simulink library "csc_rtc_rts_collection_lib"  (R2014b)
settings: Solver=ode45  StartTime=0.0  StopTime=10.0  RelTol=1e-3
libraries: csu_exr_execute_rts_lib x11, util_info_lib x1
settings Model: Creator=jimkaidy  LastModifiedBy=jimkaidy

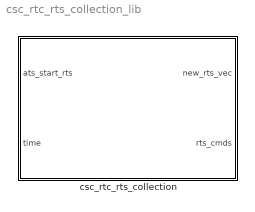
== system csc_rtc_rts_collection_lib ==
  csc_rtc_rts_collection : Subsystem
      mask Display: color('blue');text(0.05, 0.02, 'MoonEx', 'HorizontalAlignment', 'Left', 'VerticalAlignment', 'Bottom');color('red');text(0.95, 0.02, 'Autogenerated', 'HorizontalAlignment', 'Right', 'VerticalAlignment', 'Bottom');

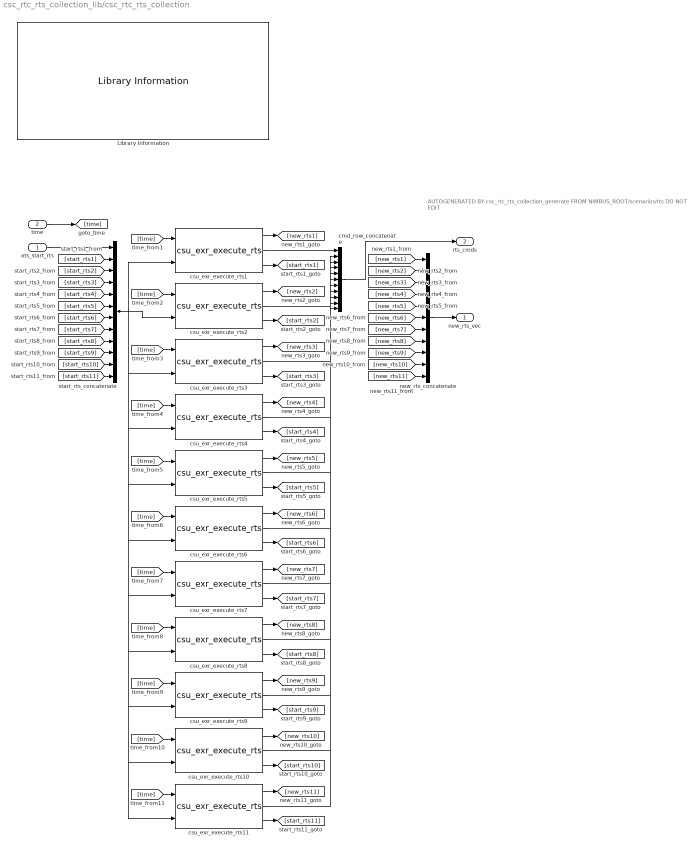
== system csc_rtc_rts_collection_lib/csc_rtc_rts_collection ==
  note: AUTOGENERATED BY csc_rtc_rts_collection_generate FROM
      | NIMBUS_ROOT/scenarios/rts
      | DO NOT EDIT
  ats_start_rts : Inport
  time : Inport  Port=2
  Library Information : util_info_lib/Library Information  owner='escrane'
  cmd_row_concatenate : Concatenate  NumInputs=11  Mode=Multidimensional array
  csu_exr_execute_rts1 : csu_exr_execute_rts_lib/csu_exr_execute_rts  rts_id=10  rts_tbl_cmd_time=sc_rts010_cmd_time  rts_tbl_cmd_data=sc_rts010_cmd_data
  csu_exr_execute_rts10 : csu_exr_execute_rts_lib/csu_exr_execute_rts  rts_id=52  rts_tbl_cmd_time=sc_rts052_cmd_time  rts_tbl_cmd_data=sc_rts052_cmd_data
  csu_exr_execute_rts11 : csu_exr_execute_rts_lib/csu_exr_execute_rts  rts_id=81  rts_tbl_cmd_time=sc_rts081_cmd_time  rts_tbl_cmd_data=sc_rts081_cmd_data
  csu_exr_execute_rts2 : csu_exr_execute_rts_lib/csu_exr_execute_rts  rts_id=12  rts_tbl_cmd_time=sc_rts012_cmd_time  rts_tbl_cmd_data=sc_rts012_cmd_data
  csu_exr_execute_rts3 : csu_exr_execute_rts_lib/csu_exr_execute_rts  rts_id=13  rts_tbl_cmd_time=sc_rts013_cmd_time  rts_tbl_cmd_data=sc_rts013_cmd_data
  csu_exr_execute_rts4 : csu_exr_execute_rts_lib/csu_exr_execute_rts  rts_id=14  rts_tbl_cmd_time=sc_rts014_cmd_time  rts_tbl_cmd_data=sc_rts014_cmd_data
  csu_exr_execute_rts5 : csu_exr_execute_rts_lib/csu_exr_execute_rts  rts_id=15  rts_tbl_cmd_time=sc_rts015_cmd_time  rts_tbl_cmd_data=sc_rts015_cmd_data
  csu_exr_execute_rts6 : csu_exr_execute_rts_lib/csu_exr_execute_rts  rts_id=1  rts_tbl_cmd_time=sc_rts001_cmd_time  rts_tbl_cmd_data=sc_rts001_cmd_data
  csu_exr_execute_rts7 : csu_exr_execute_rts_lib/csu_exr_execute_rts  rts_id=40  rts_tbl_cmd_time=sc_rts040_cmd_time  rts_tbl_cmd_data=sc_rts040_cmd_data
  csu_exr_execute_rts8 : csu_exr_execute_rts_lib/csu_exr_execute_rts  rts_id=50  rts_tbl_cmd_time=sc_rts050_cmd_time  rts_tbl_cmd_data=sc_rts050_cmd_data
  csu_exr_execute_rts9 : csu_exr_execute_rts_lib/csu_exr_execute_rts  rts_id=51  rts_tbl_cmd_time=sc_rts051_cmd_time  rts_tbl_cmd_data=sc_rts051_cmd_data
  new_rts_concatenate : Concatenate  NumInputs=11
  start_rts_concatenate : Concatenate  NumInputs=12
  new_rts_vec : Outport
  rts_cmds : Outport  Port=2
  wires:
  time/1 -> [time]
  ats_start_rts/1 -> start_rts_concatenate/1
  new_rts_concatenate/1 -> new_rts_vec/1
  [start_rts1] -> start_rts_concatenate/2
  [new_rts1] -> new_rts_concatenate/1
  [time] -> csu_exr_execute_rts1/1
  csu_exr_execute_rts1/1 -> [new_rts1]
  csu_exr_execute_rts1/3 -> [start_rts1]
  [start_rts2] -> start_rts_concatenate/3
  [new_rts2] -> new_rts_concatenate/2
  [time] -> csu_exr_execute_rts2/1
  csu_exr_execute_rts2/1 -> [new_rts2]
  csu_exr_execute_rts2/3 -> [start_rts2]
  [start_rts3] -> start_rts_concatenate/4
  [new_rts3] -> new_rts_concatenate/3
  [time] -> csu_exr_execute_rts3/1
  csu_exr_execute_rts3/1 -> [new_rts3]
  csu_exr_execute_rts3/3 -> [start_rts3]
  [start_rts4] -> start_rts_concatenate/5
  [new_rts4] -> new_rts_concatenate/4
  [time] -> csu_exr_execute_rts4/1
  csu_exr_execute_rts4/1 -> [new_rts4]
  csu_exr_execute_rts4/3 -> [start_rts4]
  [start_rts5] -> start_rts_concatenate/6
  [new_rts5] -> new_rts_concatenate/5
  [time] -> csu_exr_execute_rts5/1
  csu_exr_execute_rts5/1 -> [new_rts5]
  csu_exr_execute_rts5/3 -> [start_rts5]
  [start_rts6] -> start_rts_concatenate/7
  [new_rts6] -> new_rts_concatenate/6
  [time] -> csu_exr_execute_rts6/1
  csu_exr_execute_rts6/1 -> [new_rts6]
  csu_exr_execute_rts6/3 -> [start_rts6]
  [start_rts7] -> start_rts_concatenate/8
  [new_rts7] -> new_rts_concatenate/7
  [time] -> csu_exr_execute_rts7/1
  csu_exr_execute_rts7/1 -> [new_rts7]
  csu_exr_execute_rts7/3 -> [start_rts7]
  [start_rts8] -> start_rts_concatenate/9
  [new_rts8] -> new_rts_concatenate/8
  [time] -> csu_exr_execute_rts8/1
  csu_exr_execute_rts8/1 -> [new_rts8]
  csu_exr_execute_rts8/3 -> [start_rts8]
  [start_rts9] -> start_rts_concatenate/10
  [new_rts9] -> new_rts_concatenate/9
  [time] -> csu_exr_execute_rts9/1
  csu_exr_execute_rts9/1 -> [new_rts9]
  csu_exr_execute_rts9/3 -> [start_rts9]
  [start_rts10] -> start_rts_concatenate/11
  [new_rts10] -> new_rts_concatenate/10
  [time] -> csu_exr_execute_rts10/1
  csu_exr_execute_rts10/1 -> [new_rts10]
  csu_exr_execute_rts10/3 -> [start_rts10]
  [start_rts11] -> start_rts_concatenate/12
  [new_rts11] -> new_rts_concatenate/11
  [time] -> csu_exr_execute_rts11/1
  csu_exr_execute_rts11/1 -> [new_rts11]
  csu_exr_execute_rts11/3 -> [start_rts11]
  cmd_row_concatenate/1 -> rts_cmds/1
  start_rts_concatenate/1 -> csu_exr_execute_rts1/2, csu_exr_execute_rts2/2, csu_exr_execute_rts3/2, csu_exr_execute_rts4/2, csu_exr_execute_rts5/2, csu_exr_execute_rts6/2, csu_exr_execute_rts7/2, csu_exr_execute_rts8/2, csu_exr_execute_rts9/2, csu_exr_execute_rts10/2, csu_exr_execute_rts11/2
  csu_exr_execute_rts1/2 -> cmd_row_concatenate/1
  csu_exr_execute_rts2/2 -> cmd_row_concatenate/2
  csu_exr_execute_rts3/2 -> cmd_row_concatenate/3
  csu_exr_execute_rts4/2 -> cmd_row_concatenate/4
  csu_exr_execute_rts5/2 -> cmd_row_concatenate/5
  csu_exr_execute_rts6/2 -> cmd_row_concatenate/6
  csu_exr_execute_rts7/2 -> cmd_row_concatenate/7
  csu_exr_execute_rts8/2 -> cmd_row_concatenate/8
  csu_exr_execute_rts9/2 -> cmd_row_concatenate/9
  csu_exr_execute_rts10/2 -> cmd_row_concatenate/10
  csu_exr_execute_rts11/2 -> cmd_row_concatenate/11
